simulink model "GunnerusDP_v1"  (R2017b)
settings: Solver=ode4  StartTime=0.0  StopTime=Tsim  FixedStep=ts  RelTol=1e-3  EnableMultiTasking=on
values from neighbouring files (symbols this model uses):
  ts = 0.01    [InitGunnerusDP.m]
undefined symbols (not defined in the file or in its folder): Control, Current, Hoerner, Par, Sim, TC_currentChange, vessel, vesselABC
libraries: marine_hydro x4, marine_gnc x3, simulink x3
(part 2 of 4)

== system GunnerusDP_v1/Environment and Vessel Dynamics/Wave definiton (from MCSim)/wave height and wave frequency/Hs and omega17 ==
  t : Inport
  Mux : Mux  Inputs=2
  hs : Subsystem  mask{v1=Par.Wave.hs(17), v2=Par.Wave.hs(18), t1=Par.Wave.time_change(33), t2=Par.Wave.time_change(34)}
      mask prompts: v1 "value1"; v2 "value2"; t1 "time1"; t2 "time2"
      mask Display:
      | plot([0 1 4 5], [0 0 4 4])
      | port_label('output', 1, 'y')
      | port_label('input', 1, 'time')
  omega_p : Subsystem  mask{v1=Par.Wave.omega_peak(17), v2=Par.Wave.omega_peak(18), t1=Par.Wave.time_change(33), t2=Par.Wave.time_change(34)}
      mask prompts: v1 "value1"; v2 "value2"; t1 "time1"; t2 "time2"
      mask Display:
      | plot([0 1 4 5], [0 0 4 4])
      | port_label('output', 1, 'y')
      | port_label('input', 1, 'time')
  Hs : Outport
  Hs n omega : Outport  Port=2
  wires:
  omega_p/1(omega_peak) -> Mux/2
  Mux/1 -> Hs n omega/1
  hs/1(omega_peak) -> Mux/1, Hs/1
  t/1 -> hs/1(time), omega_p/1(time)

== system GunnerusDP_v1/Environment and Vessel Dynamics/Wave definiton (from MCSim)/wave height and wave frequency/Hs and omega18 ==
  t : Inport
  Mux : Mux  Inputs=2
  hs : Subsystem  mask{v1=Par.Wave.hs(18), v2=Par.Wave.hs(19), t1=Par.Wave.time_change(35), t2=Par.Wave.time_change(36)}
      mask prompts: v1 "value1"; v2 "value2"; t1 "time1"; t2 "time2"
      mask Display:
      | plot([0 1 4 5], [0 0 4 4])
      | port_label('output', 1, 'y')
      | port_label('input', 1, 'time')
  omega_p : Subsystem  mask{v1=Par.Wave.omega_peak(18), v2=Par.Wave.omega_peak(19), t1=Par.Wave.time_change(35), t2=Par.Wave.time_change(36)}
      mask prompts: v1 "value1"; v2 "value2"; t1 "time1"; t2 "time2"
      mask Display:
      | plot([0 1 4 5], [0 0 4 4])
      | port_label('output', 1, 'y')
      | port_label('input', 1, 'time')
  Hs : Outport
  Hs n omega : Outport  Port=2
  wires:
  t/1 -> omega_p/1(time), hs/1(time)
  hs/1(omega_peak) -> Hs/1, Mux/1
  Mux/1 -> Hs n omega/1
  omega_p/1(omega_peak) -> Mux/2

== system GunnerusDP_v1/Environment and Vessel Dynamics/Wave definiton (from MCSim)/wave height and wave frequency/Hs and omega19 ==
  t : Inport
  Mux : Mux  Inputs=2
  hs : Subsystem  mask{v1=Par.Wave.hs(19), v2=Par.Wave.hs(20), t1=Par.Wave.time_change(37), t2=Par.Wave.time_change(38)}
      mask prompts: v1 "value1"; v2 "value2"; t1 "time1"; t2 "time2"
      mask Display:
      | plot([0 1 4 5], [0 0 4 4])
      | port_label('output', 1, 'y')
      | port_label('input', 1, 'time')
  omega_p : Subsystem  mask{v1=Par.Wave.omega_peak(19), v2=Par.Wave.omega_peak(20), t1=Par.Wave.time_change(37), t2=Par.Wave.time_change(38)}
      mask prompts: v1 "value1"; v2 "value2"; t1 "time1"; t2 "time2"
      mask Display:
      | plot([0 1 4 5], [0 0 4 4])
      | port_label('output', 1, 'y')
      | port_label('input', 1, 'time')
  Hs : Outport
  Hs n omega : Outport  Port=2
  wires:
  omega_p/1(omega_peak) -> Mux/2
  Mux/1 -> Hs n omega/1
  hs/1(omega_peak) -> Mux/1, Hs/1
  t/1 -> hs/1(time), omega_p/1(time)

== system GunnerusDP_v1/Environment and Vessel Dynamics/Wave definiton (from MCSim)/wave height and wave frequency/Hs and omega2 ==
  t : Inport
  Mux : Mux  Inputs=2
  hs : Subsystem  mask{v1=Par.Wave.hs(2), v2=Par.Wave.hs(3), t1=Par.Wave.time_change(3), t2=Par.Wave.time_change(4)}
      mask prompts: v1 "value1"; v2 "value2"; t1 "time1"; t2 "time2"
      mask Display:
      | plot([0 1 4 5], [0 0 4 4])
      | port_label('output', 1, 'y')
      | port_label('input', 1, 'time')
  omega_p : Subsystem  mask{v1=Par.Wave.omega_peak(2), v2=Par.Wave.omega_peak(3), t1=Par.Wave.time_change(3), t2=Par.Wave.time_change(4)}
      mask prompts: v1 "value1"; v2 "value2"; t1 "time1"; t2 "time2"
      mask Display:
      | plot([0 1 4 5], [0 0 4 4])
      | port_label('output', 1, 'y')
      | port_label('input', 1, 'time')
  Hs : Outport
  Hs n omega : Outport  Port=2
  wires:
  omega_p/1(omega_peak) -> Mux/2
  Mux/1 -> Hs n omega/1
  hs/1(omega_peak) -> Mux/1, Hs/1
  t/1 -> hs/1(time), omega_p/1(time)

== system GunnerusDP_v1/Environment and Vessel Dynamics/Wave definiton (from MCSim)/wave height and wave frequency/Hs and omega20 ==
  t : Inport
  Mux : Mux  Inputs=2
  hs : Subsystem  mask{v1=Par.Wave.hs(20), v2=Par.Wave.hs(21), t1=Par.Wave.time_change(39), t2=Par.Wave.time_change(40)}
      mask prompts: v1 "value1"; v2 "value2"; t1 "time1"; t2 "time2"
      mask Display:
      | plot([0 1 4 5], [0 0 4 4])
      | port_label('output', 1, 'y')
      | port_label('input', 1, 'time')
  omega_p : Subsystem  mask{v1=Par.Wave.omega_peak(20), v2=Par.Wave.omega_peak(21), t1=Par.Wave.time_change(39), t2=Par.Wave.time_change(40)}
      mask prompts: v1 "value1"; v2 "value2"; t1 "time1"; t2 "time2"
      mask Display:
      | plot([0 1 4 5], [0 0 4 4])
      | port_label('output', 1, 'y')
      | port_label('input', 1, 'time')
  Hs : Outport
  Hs n omega : Outport  Port=2
  wires:
  t/1 -> omega_p/1(time), hs/1(time)
  hs/1(omega_peak) -> Hs/1, Mux/1
  Mux/1 -> Hs n omega/1
  omega_p/1(omega_peak) -> Mux/2

== system GunnerusDP_v1/Environment and Vessel Dynamics/Wave definiton (from MCSim)/wave height and wave frequency/Hs and omega21 ==
  t : Inport
  Mux : Mux  Inputs=2
  hs : Subsystem  mask{v1=Par.Wave.hs(21), v2=Par.Wave.hs(22), t1=Par.Wave.time_change(41), t2=Par.Wave.time_change(42)}
      mask prompts: v1 "value1"; v2 "value2"; t1 "time1"; t2 "time2"
      mask Display:
      | plot([0 1 4 5], [0 0 4 4])
      | port_label('output', 1, 'y')
      | port_label('input', 1, 'time')
  omega_p : Subsystem  mask{v1=Par.Wave.omega_peak(21), v2=Par.Wave.omega_peak(22), t1=Par.Wave.time_change(41), t2=Par.Wave.time_change(42)}
      mask prompts: v1 "value1"; v2 "value2"; t1 "time1"; t2 "time2"
      mask Display:
      | plot([0 1 4 5], [0 0 4 4])
      | port_label('output', 1, 'y')
      | port_label('input', 1, 'time')
  Hs : Outport
  Hs n omega : Outport  Port=2
  wires:
  omega_p/1(omega_peak) -> Mux/2
  Mux/1 -> Hs n omega/1
  hs/1(omega_peak) -> Mux/1, Hs/1
  t/1 -> hs/1(time), omega_p/1(time)

== system GunnerusDP_v1/Environment and Vessel Dynamics/Wave definiton (from MCSim)/wave height and wave frequency/Hs and omega22 ==
  t : Inport
  Mux : Mux  Inputs=2
  hs : Subsystem  mask{v1=Par.Wave.hs(22), v2=Par.Wave.hs(23), t1=Par.Wave.time_change(43), t2=Par.Wave.time_change(44)}
      mask prompts: v1 "value1"; v2 "value2"; t1 "time1"; t2 "time2"
      mask Display:
      | plot([0 1 4 5], [0 0 4 4])
      | port_label('output', 1, 'y')
      | port_label('input', 1, 'time')
  omega_p : Subsystem  mask{v1=Par.Wave.omega_peak(22), v2=Par.Wave.omega_peak(23), t1=Par.Wave.time_change(43), t2=Par.Wave.time_change(44)}
      mask prompts: v1 "value1"; v2 "value2"; t1 "time1"; t2 "time2"
      mask Display:
      | plot([0 1 4 5], [0 0 4 4])
      | port_label('output', 1, 'y')
      | port_label('input', 1, 'time')
  Hs : Outport
  Hs n omega : Outport  Port=2
  wires:
  t/1 -> omega_p/1(time), hs/1(time)
  hs/1(omega_peak) -> Hs/1, Mux/1
  Mux/1 -> Hs n omega/1
  omega_p/1(omega_peak) -> Mux/2

== system GunnerusDP_v1/Environment and Vessel Dynamics/Wave definiton (from MCSim)/wave height and wave frequency/Hs and omega23 ==
  t : Inport
  Mux : Mux  Inputs=2
  hs : Subsystem  mask{v1=Par.Wave.hs(23), v2=Par.Wave.hs(24), t1=Par.Wave.time_change(45), t2=Par.Wave.time_change(46)}
      mask prompts: v1 "value1"; v2 "value2"; t1 "time1"; t2 "time2"
      mask Display:
      | plot([0 1 4 5], [0 0 4 4])
      | port_label('output', 1, 'y')
      | port_label('input', 1, 'time')
  omega_p : Subsystem  mask{v1=Par.Wave.omega_peak(23), v2=Par.Wave.omega_peak(24), t1=Par.Wave.time_change(45), t2=Par.Wave.time_change(46)}
      mask prompts: v1 "value1"; v2 "value2"; t1 "time1"; t2 "time2"
      mask Display:
      | plot([0 1 4 5], [0 0 4 4])
      | port_label('output', 1, 'y')
      | port_label('input', 1, 'time')
  Hs : Outport
  Hs n omega : Outport  Port=2
  wires:
  omega_p/1(omega_peak) -> Mux/2
  Mux/1 -> Hs n omega/1
  hs/1(omega_peak) -> Mux/1, Hs/1
  t/1 -> hs/1(time), omega_p/1(time)

== system GunnerusDP_v1/Environment and Vessel Dynamics/Wave definiton (from MCSim)/wave height and wave frequency/Hs and omega24 ==
  t : Inport
  Mux : Mux  Inputs=2
  hs : Subsystem  mask{v1=Par.Wave.hs(24), v2=Par.Wave.hs(25), t1=Par.Wave.time_change(47), t2=Par.Wave.time_change(48)}
      mask prompts: v1 "value1"; v2 "value2"; t1 "time1"; t2 "time2"
      mask Display:
      | plot([0 1 4 5], [0 0 4 4])
      | port_label('output', 1, 'y')
      | port_label('input', 1, 'time')
  omega_p : Subsystem  mask{v1=Par.Wave.omega_peak(24), v2=Par.Wave.omega_peak(25), t1=Par.Wave.time_change(47), t2=Par.Wave.time_change(48)}
      mask prompts: v1 "value1"; v2 "value2"; t1 "time1"; t2 "time2"
      mask Display:
      | plot([0 1 4 5], [0 0 4 4])
      | port_label('output', 1, 'y')
      | port_label('input', 1, 'time')
  Hs : Outport
  Hs n omega : Outport  Port=2
  wires:
  t/1 -> omega_p/1(time), hs/1(time)
  hs/1(omega_peak) -> Hs/1, Mux/1
  Mux/1 -> Hs n omega/1
  omega_p/1(omega_peak) -> Mux/2

== system GunnerusDP_v1/Environment and Vessel Dynamics/Wave definiton (from MCSim)/wave height and wave frequency/Hs and omega3 ==
  t : Inport
  Mux : Mux  Inputs=2
  hs : Subsystem  mask{v1=Par.Wave.hs(3), v2=Par.Wave.hs(4), t1=Par.Wave.time_change(5), t2=Par.Wave.time_change(6)}
      mask prompts: v1 "value1"; v2 "value2"; t1 "time1"; t2 "time2"
      mask Display:
      | plot([0 1 4 5], [0 0 4 4])
      | port_label('output', 1, 'y')
      | port_label('input', 1, 'time')
  omega_p : Subsystem  mask{v1=Par.Wave.omega_peak(3), v2=Par.Wave.omega_peak(4), t1=Par.Wave.time_change(5), t2=Par.Wave.time_change(6)}
      mask prompts: v1 "value1"; v2 "value2"; t1 "time1"; t2 "time2"
      mask Display:
      | plot([0 1 4 5], [0 0 4 4])
      | port_label('output', 1, 'y')
      | port_label('input', 1, 'time')
  Hs : Outport
  Hs n omega : Outport  Port=2
  wires:
  t/1 -> omega_p/1(time), hs/1(time)
  hs/1(omega_peak) -> Hs/1, Mux/1
  Mux/1 -> Hs n omega/1
  omega_p/1(omega_peak) -> Mux/2

== system GunnerusDP_v1/Environment and Vessel Dynamics/Wave definiton (from MCSim)/wave height and wave frequency/Hs and omega4 ==
  t : Inport
  Mux : Mux  Inputs=2
  hs : Subsystem  mask{v1=Par.Wave.hs(4), v2=Par.Wave.hs(5), t1=Par.Wave.time_change(7), t2=Par.Wave.time_change(8)}
      mask prompts: v1 "value1"; v2 "value2"; t1 "time1"; t2 "time2"
      mask Display:
      | plot([0 1 4 5], [0 0 4 4])
      | port_label('output', 1, 'y')
      | port_label('input', 1, 'time')
  omega_p : Subsystem  mask{v1=Par.Wave.omega_peak(4), v2=Par.Wave.omega_peak(5), t1=Par.Wave.time_change(7), t2=Par.Wave.time_change(8)}
      mask prompts: v1 "value1"; v2 "value2"; t1 "time1"; t2 "time2"
      mask Display:
      | plot([0 1 4 5], [0 0 4 4])
      | port_label('output', 1, 'y')
      | port_label('input', 1, 'time')
  Hs : Outport
  Hs n omega : Outport  Port=2
  wires:
  omega_p/1(omega_peak) -> Mux/2
  Mux/1 -> Hs n omega/1
  hs/1(omega_peak) -> Mux/1, Hs/1
  t/1 -> hs/1(time), omega_p/1(time)

== system GunnerusDP_v1/Environment and Vessel Dynamics/Wave definiton (from MCSim)/wave height and wave frequency/Hs and omega5 ==
  t : Inport
  Mux : Mux  Inputs=2
  hs : Subsystem  mask{v1=Par.Wave.hs(5), v2=Par.Wave.hs(6), t1=Par.Wave.time_change(9), t2=Par.Wave.time_change(10)}
      mask prompts: v1 "value1"; v2 "value2"; t1 "time1"; t2 "time2"
      mask Display:
      | plot([0 1 4 5], [0 0 4 4])
      | port_label('output', 1, 'y')
      | port_label('input', 1, 'time')
  omega_p : Subsystem  mask{v1=Par.Wave.omega_peak(5), v2=Par.Wave.omega_peak(6), t1=Par.Wave.time_change(9), t2=Par.Wave.time_change(10)}
      mask prompts: v1 "value1"; v2 "value2"; t1 "time1"; t2 "time2"
      mask Display:
      | plot([0 1 4 5], [0 0 4 4])
      | port_label('output', 1, 'y')
      | port_label('input', 1, 'time')
  Hs : Outport
  Hs n omega : Outport  Port=2
  wires:
  t/1 -> omega_p/1(time), hs/1(time)
  hs/1(omega_peak) -> Hs/1, Mux/1
  Mux/1 -> Hs n omega/1
  omega_p/1(omega_peak) -> Mux/2

== system GunnerusDP_v1/Environment and Vessel Dynamics/Wave definiton (from MCSim)/wave height and wave frequency/Hs and omega6 ==
  t : Inport
  Mux : Mux  Inputs=2
  hs : Subsystem  mask{v1=Par.Wave.hs(6), v2=Par.Wave.hs(7), t1=Par.Wave.time_change(11), t2=Par.Wave.time_change(12)}
      mask prompts: v1 "value1"; v2 "value2"; t1 "time1"; t2 "time2"
      mask Display:
      | plot([0 1 4 5], [0 0 4 4])
      | port_label('output', 1, 'y')
      | port_label('input', 1, 'time')
  omega_p : Subsystem  mask{v1=Par.Wave.omega_peak(6), v2=Par.Wave.omega_peak(7), t1=Par.Wave.time_change(11), t2=Par.Wave.time_change(12)}
      mask prompts: v1 "value1"; v2 "value2"; t1 "time1"; t2 "time2"
      mask Display:
      | plot([0 1 4 5], [0 0 4 4])
      | port_label('output', 1, 'y')
      | port_label('input', 1, 'time')
  Hs : Outport
  Hs n omega : Outport  Port=2
  wires:
  omega_p/1(omega_peak) -> Mux/2
  Mux/1 -> Hs n omega/1
  hs/1(omega_peak) -> Mux/1, Hs/1
  t/1 -> hs/1(time), omega_p/1(time)

== system GunnerusDP_v1/Environment and Vessel Dynamics/Wave definiton (from MCSim)/wave height and wave frequency/Hs and omega7 ==
  t : Inport
  Mux : Mux  Inputs=2
  hs : Subsystem  mask{v1=Par.Wave.hs(7), v2=Par.Wave.hs(8), t1=Par.Wave.time_change(13), t2=Par.Wave.time_change(14)}
      mask prompts: v1 "value1"; v2 "value2"; t1 "time1"; t2 "time2"
      mask Display:
      | plot([0 1 4 5], [0 0 4 4])
      | port_label('output', 1, 'y')
      | port_label('input', 1, 'time')
  omega_p : Subsystem  mask{v1=Par.Wave.omega_peak(7), v2=Par.Wave.omega_peak(8), t1=Par.Wave.time_change(13), t2=Par.Wave.time_change(14)}
      mask prompts: v1 "value1"; v2 "value2"; t1 "time1"; t2 "time2"
      mask Display:
      | plot([0 1 4 5], [0 0 4 4])
      | port_label('output', 1, 'y')
      | port_label('input', 1, 'time')
  Hs : Outport
  Hs n omega : Outport  Port=2
  wires:
  t/1 -> omega_p/1(time), hs/1(time)
  hs/1(omega_peak) -> Hs/1, Mux/1
  Mux/1 -> Hs n omega/1
  omega_p/1(omega_peak) -> Mux/2

== system GunnerusDP_v1/Environment and Vessel Dynamics/Wave definiton (from MCSim)/wave height and wave frequency/Hs and omega8 ==
  t : Inport
  Mux : Mux  Inputs=2
  hs : Subsystem  mask{v1=Par.Wave.hs(8), v2=Par.Wave.hs(9), t1=Par.Wave.time_change(15), t2=Par.Wave.time_change(16)}
      mask prompts: v1 "value1"; v2 "value2"; t1 "time1"; t2 "time2"
      mask Display:
      | plot([0 1 4 5], [0 0 4 4])
      | port_label('output', 1, 'y')
      | port_label('input', 1, 'time')
  omega_p : Subsystem  mask{v1=Par.Wave.omega_peak(8), v2=Par.Wave.omega_peak(9), t1=Par.Wave.time_change(15), t2=Par.Wave.time_change(16)}
      mask prompts: v1 "value1"; v2 "value2"; t1 "time1"; t2 "time2"
      mask Display:
      | plot([0 1 4 5], [0 0 4 4])
      | port_label('output', 1, 'y')
      | port_label('input', 1, 'time')
  Hs : Outport
  Hs n omega : Outport  Port=2
  wires:
  omega_p/1(omega_peak) -> Mux/2
  Mux/1 -> Hs n omega/1
  hs/1(omega_peak) -> Mux/1, Hs/1
  t/1 -> hs/1(time), omega_p/1(time)

== system GunnerusDP_v1/Environment and Vessel Dynamics/Wave definiton (from MCSim)/wave height and wave frequency/Hs and omega9 ==
  t : Inport
  Mux : Mux  Inputs=2
  hs : Subsystem  mask{v1=Par.Wave.hs(9), v2=Par.Wave.hs(10), t1=Par.Wave.time_change(17), t2=Par.Wave.time_change(18)}
      mask prompts: v1 "value1"; v2 "value2"; t1 "time1"; t2 "time2"
      mask Display:
      | plot([0 1 4 5], [0 0 4 4])
      | port_label('output', 1, 'y')
      | port_label('input', 1, 'time')
  omega_p : Subsystem  mask{v1=Par.Wave.omega_peak(9), v2=Par.Wave.omega_peak(10), t1=Par.Wave.time_change(17), t2=Par.Wave.time_change(18)}
      mask prompts: v1 "value1"; v2 "value2"; t1 "time1"; t2 "time2"
      mask Display:
      | plot([0 1 4 5], [0 0 4 4])
      | port_label('output', 1, 'y')
      | port_label('input', 1, 'time')
  Hs : Outport
  Hs n omega : Outport  Port=2
  wires:
  t/1 -> omega_p/1(time), hs/1(time)
  hs/1(omega_peak) -> Hs/1, Mux/1
  Mux/1 -> Hs n omega/1
  omega_p/1(omega_peak) -> Mux/2

== system GunnerusDP_v1/Environment and Vessel Dynamics/Wave definiton (from MCSim)/wave height and wave frequency/Count/switch1 ==
  hs : Inport
  Constant : Constant  Value=a
  Gain : Gain  Gain=1/(b-a)  SaturateOnIntegerOverflow=on  OutDataTypeStr=Inherit: Same as input  ParamDataTypeStr=Inherit: Same as input
  Sum : Sum  Inputs=-+  SaturateOnIntegerOverflow=on
  switch : Outport
  wires:
  Constant/1 -> Sum/1
  Sum/1 -> Gain/1
  Gain/1 -> switch/1
  hs/1 -> Sum/2

== system GunnerusDP_v1/Environment and Vessel Dynamics/Wave definiton (from MCSim)/wave height and wave frequency/Count/switch10 ==
  hs : Inport
  Constant : Constant  Value=a
  Gain : Gain  Gain=1/(b-a)  SaturateOnIntegerOverflow=on  OutDataTypeStr=Inherit: Same as input  ParamDataTypeStr=Inherit: Same as input
  Sum : Sum  Inputs=-+  SaturateOnIntegerOverflow=on
  switch : Outport
  wires:
  hs/1 -> Sum/2
  Gain/1 -> switch/1
  Sum/1 -> Gain/1
  Constant/1 -> Sum/1

== system GunnerusDP_v1/Environment and Vessel Dynamics/Wave definiton (from MCSim)/wave height and wave frequency/Count/switch11 ==
  hs : Inport
  Constant : Constant  Value=a
  Gain : Gain  Gain=1/(b-a)  SaturateOnIntegerOverflow=on  OutDataTypeStr=Inherit: Same as input  ParamDataTypeStr=Inherit: Same as input
  Sum : Sum  Inputs=-+  SaturateOnIntegerOverflow=on
  switch : Outport
  wires:
  hs/1 -> Sum/2
  Gain/1 -> switch/1
  Sum/1 -> Gain/1
  Constant/1 -> Sum/1

== system GunnerusDP_v1/Environment and Vessel Dynamics/Wave definiton (from MCSim)/wave height and wave frequency/Count/switch12 ==
  hs : Inport
  Constant : Constant  Value=a
  Gain : Gain  Gain=1/(b-a)  SaturateOnIntegerOverflow=on  OutDataTypeStr=Inherit: Same as input  ParamDataTypeStr=Inherit: Same as input
  Sum : Sum  Inputs=-+  SaturateOnIntegerOverflow=on
  switch : Outport
  wires:
  hs/1 -> Sum/2
  Gain/1 -> switch/1
  Sum/1 -> Gain/1
  Constant/1 -> Sum/1

== system GunnerusDP_v1/Environment and Vessel Dynamics/Wave definiton (from MCSim)/wave height and wave frequency/Count/switch13 ==
  hs : Inport
  Constant : Constant  Value=a
  Gain : Gain  Gain=1/(b-a)  SaturateOnIntegerOverflow=on  OutDataTypeStr=Inherit: Same as input  ParamDataTypeStr=Inherit: Same as input
  Sum : Sum  Inputs=-+  SaturateOnIntegerOverflow=on
  switch : Outport
  wires:
  hs/1 -> Sum/2
  Gain/1 -> switch/1
  Sum/1 -> Gain/1
  Constant/1 -> Sum/1

== system GunnerusDP_v1/Environment and Vessel Dynamics/Wave definiton (from MCSim)/wave height and wave frequency/Count/switch14 ==
  hs : Inport
  Constant : Constant  Value=a
  Gain : Gain  Gain=1/(b-a)  SaturateOnIntegerOverflow=on  OutDataTypeStr=Inherit: Same as input  ParamDataTypeStr=Inherit: Same as input
  Sum : Sum  Inputs=-+  SaturateOnIntegerOverflow=on
  switch : Outport
  wires:
  hs/1 -> Sum/2
  Gain/1 -> switch/1
  Sum/1 -> Gain/1
  Constant/1 -> Sum/1

== system GunnerusDP_v1/Environment and Vessel Dynamics/Wave definiton (from MCSim)/wave height and wave frequency/Count/switch15 ==
  hs : Inport
  Constant : Constant  Value=a
  Gain : Gain  Gain=1/(b-a)  SaturateOnIntegerOverflow=on  OutDataTypeStr=Inherit: Same as input  ParamDataTypeStr=Inherit: Same as input
  Sum : Sum  Inputs=-+  SaturateOnIntegerOverflow=on
  switch : Outport
  wires:
  hs/1 -> Sum/2
  Gain/1 -> switch/1
  Sum/1 -> Gain/1
  Constant/1 -> Sum/1

== system GunnerusDP_v1/Environment and Vessel Dynamics/Wave definiton (from MCSim)/wave height and wave frequency/Count/switch16 ==
  hs : Inport
  Constant : Constant  Value=a
  Gain : Gain  Gain=1/(b-a)  SaturateOnIntegerOverflow=on  OutDataTypeStr=Inherit: Same as input  ParamDataTypeStr=Inherit: Same as input
  Sum : Sum  Inputs=-+  SaturateOnIntegerOverflow=on
  switch : Outport
  wires:
  hs/1 -> Sum/2
  Gain/1 -> switch/1
  Sum/1 -> Gain/1
  Constant/1 -> Sum/1

== system GunnerusDP_v1/Environment and Vessel Dynamics/Wave definiton (from MCSim)/wave height and wave frequency/Count/switch17 ==
  hs : Inport
  Constant : Constant  Value=a
  Gain : Gain  Gain=1/(b-a)  SaturateOnIntegerOverflow=on  OutDataTypeStr=Inherit: Same as input  ParamDataTypeStr=Inherit: Same as input
  Sum : Sum  Inputs=-+  SaturateOnIntegerOverflow=on
  switch : Outport
  wires:
  Constant/1 -> Sum/1
  Sum/1 -> Gain/1
  Gain/1 -> switch/1
  hs/1 -> Sum/2

== system GunnerusDP_v1/Environment and Vessel Dynamics/Wave definiton (from MCSim)/wave height and wave frequency/Count/switch18 ==
  hs : Inport
  Constant : Constant  Value=a
  Gain : Gain  Gain=1/(b-a)  SaturateOnIntegerOverflow=on  OutDataTypeStr=Inherit: Same as input  ParamDataTypeStr=Inherit: Same as input
  Sum : Sum  Inputs=-+  SaturateOnIntegerOverflow=on
  switch : Outport
  wires:
  hs/1 -> Sum/2
  Gain/1 -> switch/1
  Sum/1 -> Gain/1
  Constant/1 -> Sum/1

== system GunnerusDP_v1/Environment and Vessel Dynamics/Wave definiton (from MCSim)/wave height and wave frequency/Count/switch19 ==
  hs : Inport
  Constant : Constant  Value=a
  Gain : Gain  Gain=1/(b-a)  SaturateOnIntegerOverflow=on  OutDataTypeStr=Inherit: Same as input  ParamDataTypeStr=Inherit: Same as input
  Sum : Sum  Inputs=-+  SaturateOnIntegerOverflow=on
  switch : Outport
  wires:
  hs/1 -> Sum/2
  Gain/1 -> switch/1
  Sum/1 -> Gain/1
  Constant/1 -> Sum/1

== system GunnerusDP_v1/Environment and Vessel Dynamics/Wave definiton (from MCSim)/wave height and wave frequency/Count/switch2 ==
  hs : Inport
  Constant : Constant  Value=a
  Gain : Gain  Gain=1/(b-a)  SaturateOnIntegerOverflow=on  OutDataTypeStr=Inherit: Same as input  ParamDataTypeStr=Inherit: Same as input
  Sum : Sum  Inputs=-+  SaturateOnIntegerOverflow=on
  switch : Outport
  wires:
  hs/1 -> Sum/2
  Gain/1 -> switch/1
  Sum/1 -> Gain/1
  Constant/1 -> Sum/1

== system GunnerusDP_v1/Environment and Vessel Dynamics/Wave definiton (from MCSim)/wave height and wave frequency/Count/switch20 ==
  hs : Inport
  Constant : Constant  Value=a
  Gain : Gain  Gain=1/(b-a)  SaturateOnIntegerOverflow=on  OutDataTypeStr=Inherit: Same as input  ParamDataTypeStr=Inherit: Same as input
  Sum : Sum  Inputs=-+  SaturateOnIntegerOverflow=on
  switch : Outport
  wires:
  hs/1 -> Sum/2
  Gain/1 -> switch/1
  Sum/1 -> Gain/1
  Constant/1 -> Sum/1

== system GunnerusDP_v1/Environment and Vessel Dynamics/Wave definiton (from MCSim)/wave height and wave frequency/Count/switch21 ==
  hs : Inport
  Constant : Constant  Value=a
  Gain : Gain  Gain=1/(b-a)  SaturateOnIntegerOverflow=on  OutDataTypeStr=Inherit: Same as input  ParamDataTypeStr=Inherit: Same as input
  Sum : Sum  Inputs=-+  SaturateOnIntegerOverflow=on
  switch : Outport
  wires:
  hs/1 -> Sum/2
  Gain/1 -> switch/1
  Sum/1 -> Gain/1
  Constant/1 -> Sum/1

== system GunnerusDP_v1/Environment and Vessel Dynamics/Wave definiton (from MCSim)/wave height and wave frequency/Count/switch22 ==
  hs : Inport
  Constant : Constant  Value=a
  Gain : Gain  Gain=1/(b-a)  SaturateOnIntegerOverflow=on  OutDataTypeStr=Inherit: Same as input  ParamDataTypeStr=Inherit: Same as input
  Sum : Sum  Inputs=-+  SaturateOnIntegerOverflow=on
  switch : Outport
  wires:
  hs/1 -> Sum/2
  Gain/1 -> switch/1
  Sum/1 -> Gain/1
  Constant/1 -> Sum/1

== system GunnerusDP_v1/Environment and Vessel Dynamics/Wave definiton (from MCSim)/wave height and wave frequency/Count/switch23 ==
  hs : Inport
  Constant : Constant  Value=a
  Gain : Gain  Gain=1/(b-a)  SaturateOnIntegerOverflow=on  OutDataTypeStr=Inherit: Same as input  ParamDataTypeStr=Inherit: Same as input
  Sum : Sum  Inputs=-+  SaturateOnIntegerOverflow=on
  switch : Outport
  wires:
  hs/1 -> Sum/2
  Gain/1 -> switch/1
  Sum/1 -> Gain/1
  Constant/1 -> Sum/1

== system GunnerusDP_v1/Environment and Vessel Dynamics/Wave definiton (from MCSim)/wave height and wave frequency/Count/switch3 ==
  hs : Inport
  Constant : Constant  Value=a
  Gain : Gain  Gain=1/(b-a)  SaturateOnIntegerOverflow=on  OutDataTypeStr=Inherit: Same as input  ParamDataTypeStr=Inherit: Same as input
  Sum : Sum  Inputs=-+  SaturateOnIntegerOverflow=on
  switch : Outport
  wires:
  hs/1 -> Sum/2
  Gain/1 -> switch/1
  Sum/1 -> Gain/1
  Constant/1 -> Sum/1

== system GunnerusDP_v1/Environment and Vessel Dynamics/Wave definiton (from MCSim)/wave height and wave frequency/Count/switch4 ==
  hs : Inport
  Constant : Constant  Value=a
  Gain : Gain  Gain=1/(b-a)  SaturateOnIntegerOverflow=on  OutDataTypeStr=Inherit: Same as input  ParamDataTypeStr=Inherit: Same as input
  Sum : Sum  Inputs=-+  SaturateOnIntegerOverflow=on
  switch : Outport
  wires:
  hs/1 -> Sum/2
  Gain/1 -> switch/1
  Sum/1 -> Gain/1
  Constant/1 -> Sum/1

== system GunnerusDP_v1/Environment and Vessel Dynamics/Wave definiton (from MCSim)/wave height and wave frequency/Count/switch5 ==
  hs : Inport
  Constant : Constant  Value=a
  Gain : Gain  Gain=1/(b-a)  SaturateOnIntegerOverflow=on  OutDataTypeStr=Inherit: Same as input  ParamDataTypeStr=Inherit: Same as input
  Sum : Sum  Inputs=-+  SaturateOnIntegerOverflow=on
  switch : Outport
  wires:
  hs/1 -> Sum/2
  Gain/1 -> switch/1
  Sum/1 -> Gain/1
  Constant/1 -> Sum/1

== system GunnerusDP_v1/Environment and Vessel Dynamics/Wave definiton (from MCSim)/wave height and wave frequency/Count/switch6 ==
  hs : Inport
  Constant : Constant  Value=a
  Gain : Gain  Gain=1/(b-a)  SaturateOnIntegerOverflow=on  OutDataTypeStr=Inherit: Same as input  ParamDataTypeStr=Inherit: Same as input
  Sum : Sum  Inputs=-+  SaturateOnIntegerOverflow=on
  switch : Outport
  wires:
  hs/1 -> Sum/2
  Gain/1 -> switch/1
  Sum/1 -> Gain/1
  Constant/1 -> Sum/1

== system GunnerusDP_v1/Environment and Vessel Dynamics/Wave definiton (from MCSim)/wave height and wave frequency/Count/switch7 ==
  hs : Inport
  Constant : Constant  Value=a
  Gain : Gain  Gain=1/(b-a)  SaturateOnIntegerOverflow=on  OutDataTypeStr=Inherit: Same as input  ParamDataTypeStr=Inherit: Same as input
  Sum : Sum  Inputs=-+  SaturateOnIntegerOverflow=on
  switch : Outport
  wires:
  hs/1 -> Sum/2
  Gain/1 -> switch/1
  Sum/1 -> Gain/1
  Constant/1 -> Sum/1

== system GunnerusDP_v1/Environment and Vessel Dynamics/Wave definiton (from MCSim)/wave height and wave frequency/Count/switch8 ==
  hs : Inport
  Constant : Constant  Value=a
  Gain : Gain  Gain=1/(b-a)  SaturateOnIntegerOverflow=on  OutDataTypeStr=Inherit: Same as input  ParamDataTypeStr=Inherit: Same as input
  Sum : Sum  Inputs=-+  SaturateOnIntegerOverflow=on
  switch : Outport
  wires:
  hs/1 -> Sum/2
  Gain/1 -> switch/1
  Sum/1 -> Gain/1
  Constant/1 -> Sum/1

== system GunnerusDP_v1/Environment and Vessel Dynamics/Wave definiton (from MCSim)/wave height and wave frequency/Count/switch9 ==
  hs : Inport
  Constant : Constant  Value=a
  Gain : Gain  Gain=1/(b-a)  SaturateOnIntegerOverflow=on  OutDataTypeStr=Inherit: Same as input  ParamDataTypeStr=Inherit: Same as input
  Sum : Sum  Inputs=-+  SaturateOnIntegerOverflow=on
  switch : Outport
  wires:
  Constant/1 -> Sum/1
  Sum/1 -> Gain/1
  Gain/1 -> switch/1
  hs/1 -> Sum/2

== system GunnerusDP_v1/Environment and Vessel Dynamics/Wave definiton (from MCSim)/wave height and wave frequency/Hs and omega1/hs ==
  time : Inport
  Constant : Constant  Value=v1
  Constant2 : Constant  Value=v2
  If : If  IfExpression=u1 < t1  ElseIfExpressions=u1>=t1 & u1<t2
  If Action Subsystem1 : Subsystem  TreatAsAtomicUnit=on
  If Action Subsystem2 : Subsystem  TreatAsAtomicUnit=on
  If Action Subsystem3 : Subsystem  TreatAsAtomicUnit=on
  Merge : Merge  Inputs=3
  omega_peak : Outport
  wires:
  time/1 -> If Action Subsystem2/1(In1), If/1
  If/3 -> If Action Subsystem3/Action
  If/1 -> If Action Subsystem1/Action
  Constant/1 -> If Action Subsystem1/1(In1)
  Constant2/1 -> If Action Subsystem3/1(In1)
  If Action Subsystem3/1(Out1) -> Merge/3
  If Action Subsystem2/1(Out1) -> Merge/2
  If/2 -> If Action Subsystem2/Action
  If Action Subsystem1/1(Out1) -> Merge/1
  Merge/1 -> omega_peak/1

== system GunnerusDP_v1/Environment and Vessel Dynamics/Wave definiton (from MCSim)/wave height and wave frequency/Hs and omega1/omega_p ==
  time : Inport
  Constant : Constant  Value=v1
  Constant2 : Constant  Value=v2
  If : If  IfExpression=u1 < t1  ElseIfExpressions=u1>=t1 & u1<t2
  If Action Subsystem1 : Subsystem  TreatAsAtomicUnit=on
  If Action Subsystem2 : Subsystem  TreatAsAtomicUnit=on
  If Action Subsystem3 : Subsystem  TreatAsAtomicUnit=on
  Merge : Merge  Inputs=3
  omega_peak : Outport
  wires:
  Merge/1 -> omega_peak/1
  If Action Subsystem1/1(Out1) -> Merge/1
  If/2 -> If Action Subsystem2/Action
  If Action Subsystem2/1(Out1) -> Merge/2
  If Action Subsystem3/1(Out1) -> Merge/3
  Constant2/1 -> If Action Subsystem3/1(In1)
  Constant/1 -> If Action Subsystem1/1(In1)
  If/1 -> If Action Subsystem1/Action
  If/3 -> If Action Subsystem3/Action
  time/1 -> If/1, If Action Subsystem2/1(In1)

== system GunnerusDP_v1/Environment and Vessel Dynamics/Wave definiton (from MCSim)/wave height and wave frequency/Hs and omega10/hs ==
  time : Inport
  Constant : Constant  Value=v1
  Constant2 : Constant  Value=v2
  If : If  IfExpression=u1 < t1  ElseIfExpressions=u1>=t1 & u1<t2
  If Action Subsystem1 : Subsystem  TreatAsAtomicUnit=on
  If Action Subsystem2 : Subsystem  TreatAsAtomicUnit=on
  If Action Subsystem3 : Subsystem  TreatAsAtomicUnit=on
  Merge : Merge  Inputs=3
  omega_peak : Outport
  wires:
  Merge/1 -> omega_peak/1
  If Action Subsystem1/1(Out1) -> Merge/1
  If/2 -> If Action Subsystem2/Action
  If Action Subsystem2/1(Out1) -> Merge/2
  If Action Subsystem3/1(Out1) -> Merge/3
  Constant2/1 -> If Action Subsystem3/1(In1)
  Constant/1 -> If Action Subsystem1/1(In1)
  If/1 -> If Action Subsystem1/Action
  If/3 -> If Action Subsystem3/Action
  time/1 -> If/1, If Action Subsystem2/1(In1)

== system GunnerusDP_v1/Environment and Vessel Dynamics/Wave definiton (from MCSim)/wave height and wave frequency/Hs and omega10/omega_p ==
  time : Inport
  Constant : Constant  Value=v1
  Constant2 : Constant  Value=v2
  If : If  IfExpression=u1 < t1  ElseIfExpressions=u1>=t1 & u1<t2
  If Action Subsystem1 : Subsystem  TreatAsAtomicUnit=on
  If Action Subsystem2 : Subsystem  TreatAsAtomicUnit=on
  If Action Subsystem3 : Subsystem  TreatAsAtomicUnit=on
  Merge : Merge  Inputs=3
  omega_peak : Outport
  wires:
  time/1 -> If Action Subsystem2/1(In1), If/1
  If/3 -> If Action Subsystem3/Action
  If/1 -> If Action Subsystem1/Action
  Constant/1 -> If Action Subsystem1/1(In1)
  Constant2/1 -> If Action Subsystem3/1(In1)
  If Action Subsystem3/1(Out1) -> Merge/3
  If Action Subsystem2/1(Out1) -> Merge/2
  If/2 -> If Action Subsystem2/Action
  If Action Subsystem1/1(Out1) -> Merge/1
  Merge/1 -> omega_peak/1

== system GunnerusDP_v1/Environment and Vessel Dynamics/Wave definiton (from MCSim)/wave height and wave frequency/Hs and omega11/hs ==
  time : Inport
  Constant : Constant  Value=v1
  Constant2 : Constant  Value=v2
  If : If  IfExpression=u1 < t1  ElseIfExpressions=u1>=t1 & u1<t2
  If Action Subsystem1 : Subsystem  TreatAsAtomicUnit=on
  If Action Subsystem2 : Subsystem  TreatAsAtomicUnit=on
  If Action Subsystem3 : Subsystem  TreatAsAtomicUnit=on
  Merge : Merge  Inputs=3
  omega_peak : Outport
  wires:
  time/1 -> If Action Subsystem2/1(In1), If/1
  If/3 -> If Action Subsystem3/Action
  If/1 -> If Action Subsystem1/Action
  Constant/1 -> If Action Subsystem1/1(In1)
  Constant2/1 -> If Action Subsystem3/1(In1)
  If Action Subsystem3/1(Out1) -> Merge/3
  If Action Subsystem2/1(Out1) -> Merge/2
  If/2 -> If Action Subsystem2/Action
  If Action Subsystem1/1(Out1) -> Merge/1
  Merge/1 -> omega_peak/1

== system GunnerusDP_v1/Environment and Vessel Dynamics/Wave definiton (from MCSim)/wave height and wave frequency/Hs and omega11/omega_p ==
  time : Inport
  Constant : Constant  Value=v1
  Constant2 : Constant  Value=v2
  If : If  IfExpression=u1 < t1  ElseIfExpressions=u1>=t1 & u1<t2
  If Action Subsystem1 : Subsystem  TreatAsAtomicUnit=on
  If Action Subsystem2 : Subsystem  TreatAsAtomicUnit=on
  If Action Subsystem3 : Subsystem  TreatAsAtomicUnit=on
  Merge : Merge  Inputs=3
  omega_peak : Outport
  wires:
  Merge/1 -> omega_peak/1
  If Action Subsystem1/1(Out1) -> Merge/1
  If/2 -> If Action Subsystem2/Action
  If Action Subsystem2/1(Out1) -> Merge/2
  If Action Subsystem3/1(Out1) -> Merge/3
  Constant2/1 -> If Action Subsystem3/1(In1)
  Constant/1 -> If Action Subsystem1/1(In1)
  If/1 -> If Action Subsystem1/Action
  If/3 -> If Action Subsystem3/Action
  time/1 -> If/1, If Action Subsystem2/1(In1)

== system GunnerusDP_v1/Environment and Vessel Dynamics/Wave definiton (from MCSim)/wave height and wave frequency/Hs and omega12/hs ==
  time : Inport
  Constant : Constant  Value=v1
  Constant2 : Constant  Value=v2
  If : If  IfExpression=u1 < t1  ElseIfExpressions=u1>=t1 & u1<t2
  If Action Subsystem1 : Subsystem  TreatAsAtomicUnit=on
  If Action Subsystem2 : Subsystem  TreatAsAtomicUnit=on
  If Action Subsystem3 : Subsystem  TreatAsAtomicUnit=on
  Merge : Merge  Inputs=3
  omega_peak : Outport
  wires:
  Merge/1 -> omega_peak/1
  If Action Subsystem1/1(Out1) -> Merge/1
  If/2 -> If Action Subsystem2/Action
  If Action Subsystem2/1(Out1) -> Merge/2
  If Action Subsystem3/1(Out1) -> Merge/3
  Constant2/1 -> If Action Subsystem3/1(In1)
  Constant/1 -> If Action Subsystem1/1(In1)
  If/1 -> If Action Subsystem1/Action
  If/3 -> If Action Subsystem3/Action
  time/1 -> If/1, If Action Subsystem2/1(In1)

== system GunnerusDP_v1/Environment and Vessel Dynamics/Wave definiton (from MCSim)/wave height and wave frequency/Hs and omega12/omega_p ==
  time : Inport
  Constant : Constant  Value=v1
  Constant2 : Constant  Value=v2
  If : If  IfExpression=u1 < t1  ElseIfExpressions=u1>=t1 & u1<t2
  If Action Subsystem1 : Subsystem  TreatAsAtomicUnit=on
  If Action Subsystem2 : Subsystem  TreatAsAtomicUnit=on
  If Action Subsystem3 : Subsystem  TreatAsAtomicUnit=on
  Merge : Merge  Inputs=3
  omega_peak : Outport
  wires:
  time/1 -> If Action Subsystem2/1(In1), If/1
  If/3 -> If Action Subsystem3/Action
  If/1 -> If Action Subsystem1/Action
  Constant/1 -> If Action Subsystem1/1(In1)
  Constant2/1 -> If Action Subsystem3/1(In1)
  If Action Subsystem3/1(Out1) -> Merge/3
  If Action Subsystem2/1(Out1) -> Merge/2
  If/2 -> If Action Subsystem2/Action
  If Action Subsystem1/1(Out1) -> Merge/1
  Merge/1 -> omega_peak/1

== system GunnerusDP_v1/Environment and Vessel Dynamics/Wave definiton (from MCSim)/wave height and wave frequency/Hs and omega13/hs ==
  time : Inport
  Constant : Constant  Value=v1
  Constant2 : Constant  Value=v2
  If : If  IfExpression=u1 < t1  ElseIfExpressions=u1>=t1 & u1<t2
  If Action Subsystem1 : Subsystem  TreatAsAtomicUnit=on
  If Action Subsystem2 : Subsystem  TreatAsAtomicUnit=on
  If Action Subsystem3 : Subsystem  TreatAsAtomicUnit=on
  Merge : Merge  Inputs=3
  omega_peak : Outport
  wires:
  time/1 -> If Action Subsystem2/1(In1), If/1
  If/3 -> If Action Subsystem3/Action
  If/1 -> If Action Subsystem1/Action
  Constant/1 -> If Action Subsystem1/1(In1)
  Constant2/1 -> If Action Subsystem3/1(In1)
  If Action Subsystem3/1(Out1) -> Merge/3
  If Action Subsystem2/1(Out1) -> Merge/2
  If/2 -> If Action Subsystem2/Action
  If Action Subsystem1/1(Out1) -> Merge/1
  Merge/1 -> omega_peak/1

== system GunnerusDP_v1/Environment and Vessel Dynamics/Wave definiton (from MCSim)/wave height and wave frequency/Hs and omega13/omega_p ==
  time : Inport
  Constant : Constant  Value=v1
  Constant2 : Constant  Value=v2
  If : If  IfExpression=u1 < t1  ElseIfExpressions=u1>=t1 & u1<t2
  If Action Subsystem1 : Subsystem  TreatAsAtomicUnit=on
  If Action Subsystem2 : Subsystem  TreatAsAtomicUnit=on
  If Action Subsystem3 : Subsystem  TreatAsAtomicUnit=on
  Merge : Merge  Inputs=3
  omega_peak : Outport
  wires:
  Merge/1 -> omega_peak/1
  If Action Subsystem1/1(Out1) -> Merge/1
  If/2 -> If Action Subsystem2/Action
  If Action Subsystem2/1(Out1) -> Merge/2
  If Action Subsystem3/1(Out1) -> Merge/3
  Constant2/1 -> If Action Subsystem3/1(In1)
  Constant/1 -> If Action Subsystem1/1(In1)
  If/1 -> If Action Subsystem1/Action
  If/3 -> If Action Subsystem3/Action
  time/1 -> If/1, If Action Subsystem2/1(In1)

== system GunnerusDP_v1/Environment and Vessel Dynamics/Wave definiton (from MCSim)/wave height and wave frequency/Hs and omega14/hs ==
  time : Inport
  Constant : Constant  Value=v1
  Constant2 : Constant  Value=v2
  If : If  IfExpression=u1 < t1  ElseIfExpressions=u1>=t1 & u1<t2
  If Action Subsystem1 : Subsystem  TreatAsAtomicUnit=on
  If Action Subsystem2 : Subsystem  TreatAsAtomicUnit=on
  If Action Subsystem3 : Subsystem  TreatAsAtomicUnit=on
  Merge : Merge  Inputs=3
  omega_peak : Outport
  wires:
  Merge/1 -> omega_peak/1
  If Action Subsystem1/1(Out1) -> Merge/1
  If/2 -> If Action Subsystem2/Action
  If Action Subsystem2/1(Out1) -> Merge/2
  If Action Subsystem3/1(Out1) -> Merge/3
  Constant2/1 -> If Action Subsystem3/1(In1)
  Constant/1 -> If Action Subsystem1/1(In1)
  If/1 -> If Action Subsystem1/Action
  If/3 -> If Action Subsystem3/Action
  time/1 -> If/1, If Action Subsystem2/1(In1)

== system GunnerusDP_v1/Environment and Vessel Dynamics/Wave definiton (from MCSim)/wave height and wave frequency/Hs and omega14/omega_p ==
  time : Inport
  Constant : Constant  Value=v1
  Constant2 : Constant  Value=v2
  If : If  IfExpression=u1 < t1  ElseIfExpressions=u1>=t1 & u1<t2
  If Action Subsystem1 : Subsystem  TreatAsAtomicUnit=on
  If Action Subsystem2 : Subsystem  TreatAsAtomicUnit=on
  If Action Subsystem3 : Subsystem  TreatAsAtomicUnit=on
  Merge : Merge  Inputs=3
  omega_peak : Outport
  wires:
  time/1 -> If Action Subsystem2/1(In1), If/1
  If/3 -> If Action Subsystem3/Action
  If/1 -> If Action Subsystem1/Action
  Constant/1 -> If Action Subsystem1/1(In1)
  Constant2/1 -> If Action Subsystem3/1(In1)
  If Action Subsystem3/1(Out1) -> Merge/3
  If Action Subsystem2/1(Out1) -> Merge/2
  If/2 -> If Action Subsystem2/Action
  If Action Subsystem1/1(Out1) -> Merge/1
  Merge/1 -> omega_peak/1

== system GunnerusDP_v1/Environment and Vessel Dynamics/Wave definiton (from MCSim)/wave height and wave frequency/Hs and omega15/hs ==
  time : Inport
  Constant : Constant  Value=v1
  Constant2 : Constant  Value=v2
  If : If  IfExpression=u1 < t1  ElseIfExpressions=u1>=t1 & u1<t2
  If Action Subsystem1 : Subsystem  TreatAsAtomicUnit=on
  If Action Subsystem2 : Subsystem  TreatAsAtomicUnit=on
  If Action Subsystem3 : Subsystem  TreatAsAtomicUnit=on
  Merge : Merge  Inputs=3
  omega_peak : Outport
  wires:
  time/1 -> If Action Subsystem2/1(In1), If/1
  If/3 -> If Action Subsystem3/Action
  If/1 -> If Action Subsystem1/Action
  Constant/1 -> If Action Subsystem1/1(In1)
  Constant2/1 -> If Action Subsystem3/1(In1)
  If Action Subsystem3/1(Out1) -> Merge/3
  If Action Subsystem2/1(Out1) -> Merge/2
  If/2 -> If Action Subsystem2/Action
  If Action Subsystem1/1(Out1) -> Merge/1
  Merge/1 -> omega_peak/1

== system GunnerusDP_v1/Environment and Vessel Dynamics/Wave definiton (from MCSim)/wave height and wave frequency/Hs and omega15/omega_p ==
  time : Inport
  Constant : Constant  Value=v1
  Constant2 : Constant  Value=v2
  If : If  IfExpression=u1 < t1  ElseIfExpressions=u1>=t1 & u1<t2
  If Action Subsystem1 : Subsystem  TreatAsAtomicUnit=on
  If Action Subsystem2 : Subsystem  TreatAsAtomicUnit=on
  If Action Subsystem3 : Subsystem  TreatAsAtomicUnit=on
  Merge : Merge  Inputs=3
  omega_peak : Outport
  wires:
  Merge/1 -> omega_peak/1
  If Action Subsystem1/1(Out1) -> Merge/1
  If/2 -> If Action Subsystem2/Action
  If Action Subsystem2/1(Out1) -> Merge/2
  If Action Subsystem3/1(Out1) -> Merge/3
  Constant2/1 -> If Action Subsystem3/1(In1)
  Constant/1 -> If Action Subsystem1/1(In1)
  If/1 -> If Action Subsystem1/Action
  If/3 -> If Action Subsystem3/Action
  time/1 -> If/1, If Action Subsystem2/1(In1)

== system GunnerusDP_v1/Environment and Vessel Dynamics/Wave definiton (from MCSim)/wave height and wave frequency/Hs and omega16/hs ==
  time : Inport
  Constant : Constant  Value=v1
  Constant2 : Constant  Value=v2
  If : If  IfExpression=u1 < t1  ElseIfExpressions=u1>=t1 & u1<t2
  If Action Subsystem1 : Subsystem  TreatAsAtomicUnit=on
  If Action Subsystem2 : Subsystem  TreatAsAtomicUnit=on
  If Action Subsystem3 : Subsystem  TreatAsAtomicUnit=on
  Merge : Merge  Inputs=3
  omega_peak : Outport
  wires:
  time/1 -> If Action Subsystem2/1(In1), If/1
  If/3 -> If Action Subsystem3/Action
  If/1 -> If Action Subsystem1/Action
  Constant/1 -> If Action Subsystem1/1(In1)
  Constant2/1 -> If Action Subsystem3/1(In1)
  If Action Subsystem3/1(Out1) -> Merge/3
  If Action Subsystem2/1(Out1) -> Merge/2
  If/2 -> If Action Subsystem2/Action
  If Action Subsystem1/1(Out1) -> Merge/1
  Merge/1 -> omega_peak/1

== system GunnerusDP_v1/Environment and Vessel Dynamics/Wave definiton (from MCSim)/wave height and wave frequency/Hs and omega16/omega_p ==
  time : Inport
  Constant : Constant  Value=v1
  Constant2 : Constant  Value=v2
  If : If  IfExpression=u1 < t1  ElseIfExpressions=u1>=t1 & u1<t2
  If Action Subsystem1 : Subsystem  TreatAsAtomicUnit=on
  If Action Subsystem2 : Subsystem  TreatAsAtomicUnit=on
  If Action Subsystem3 : Subsystem  TreatAsAtomicUnit=on
  Merge : Merge  Inputs=3
  omega_peak : Outport
  wires:
  Merge/1 -> omega_peak/1
  If Action Subsystem1/1(Out1) -> Merge/1
  If/2 -> If Action Subsystem2/Action
  If Action Subsystem2/1(Out1) -> Merge/2
  If Action Subsystem3/1(Out1) -> Merge/3
  Constant2/1 -> If Action Subsystem3/1(In1)
  Constant/1 -> If Action Subsystem1/1(In1)
  If/1 -> If Action Subsystem1/Action
  If/3 -> If Action Subsystem3/Action
  time/1 -> If/1, If Action Subsystem2/1(In1)

== system GunnerusDP_v1/Environment and Vessel Dynamics/Wave definiton (from MCSim)/wave height and wave frequency/Hs and omega17/hs ==
  time : Inport
  Constant : Constant  Value=v1
  Constant2 : Constant  Value=v2
  If : If  IfExpression=u1 < t1  ElseIfExpressions=u1>=t1 & u1<t2
  If Action Subsystem1 : Subsystem  TreatAsAtomicUnit=on
  If Action Subsystem2 : Subsystem  TreatAsAtomicUnit=on
  If Action Subsystem3 : Subsystem  TreatAsAtomicUnit=on
  Merge : Merge  Inputs=3
  omega_peak : Outport
  wires:
  Merge/1 -> omega_peak/1
  If Action Subsystem1/1(Out1) -> Merge/1
  If/2 -> If Action Subsystem2/Action
  If Action Subsystem2/1(Out1) -> Merge/2
  If Action Subsystem3/1(Out1) -> Merge/3
  Constant2/1 -> If Action Subsystem3/1(In1)
  Constant/1 -> If Action Subsystem1/1(In1)
  If/1 -> If Action Subsystem1/Action
  If/3 -> If Action Subsystem3/Action
  time/1 -> If/1, If Action Subsystem2/1(In1)

== system GunnerusDP_v1/Environment and Vessel Dynamics/Wave definiton (from MCSim)/wave height and wave frequency/Hs and omega17/omega_p ==
  time : Inport
  Constant : Constant  Value=v1
  Constant2 : Constant  Value=v2
  If : If  IfExpression=u1 < t1  ElseIfExpressions=u1>=t1 & u1<t2
  If Action Subsystem1 : Subsystem  TreatAsAtomicUnit=on
  If Action Subsystem2 : Subsystem  TreatAsAtomicUnit=on
  If Action Subsystem3 : Subsystem  TreatAsAtomicUnit=on
  Merge : Merge  Inputs=3
  omega_peak : Outport
  wires:
  time/1 -> If Action Subsystem2/1(In1), If/1
  If/3 -> If Action Subsystem3/Action
  If/1 -> If Action Subsystem1/Action
  Constant/1 -> If Action Subsystem1/1(In1)
  Constant2/1 -> If Action Subsystem3/1(In1)
  If Action Subsystem3/1(Out1) -> Merge/3
  If Action Subsystem2/1(Out1) -> Merge/2
  If/2 -> If Action Subsystem2/Action
  If Action Subsystem1/1(Out1) -> Merge/1
  Merge/1 -> omega_peak/1

== system GunnerusDP_v1/Environment and Vessel Dynamics/Wave definiton (from MCSim)/wave height and wave frequency/Hs and omega18/hs ==
  time : Inport
  Constant : Constant  Value=v1
  Constant2 : Constant  Value=v2
  If : If  IfExpression=u1 < t1  ElseIfExpressions=u1>=t1 & u1<t2
  If Action Subsystem1 : Subsystem  TreatAsAtomicUnit=on
  If Action Subsystem2 : Subsystem  TreatAsAtomicUnit=on
  If Action Subsystem3 : Subsystem  TreatAsAtomicUnit=on
  Merge : Merge  Inputs=3
  omega_peak : Outport
  wires:
  time/1 -> If Action Subsystem2/1(In1), If/1
  If/3 -> If Action Subsystem3/Action
  If/1 -> If Action Subsystem1/Action
  Constant/1 -> If Action Subsystem1/1(In1)
  Constant2/1 -> If Action Subsystem3/1(In1)
  If Action Subsystem3/1(Out1) -> Merge/3
  If Action Subsystem2/1(Out1) -> Merge/2
  If/2 -> If Action Subsystem2/Action
  If Action Subsystem1/1(Out1) -> Merge/1
  Merge/1 -> omega_peak/1

== system GunnerusDP_v1/Environment and Vessel Dynamics/Wave definiton (from MCSim)/wave height and wave frequency/Hs and omega18/omega_p ==
  time : Inport
  Constant : Constant  Value=v1
  Constant2 : Constant  Value=v2
  If : If  IfExpression=u1 < t1  ElseIfExpressions=u1>=t1 & u1<t2
  If Action Subsystem1 : Subsystem  TreatAsAtomicUnit=on
  If Action Subsystem2 : Subsystem  TreatAsAtomicUnit=on
  If Action Subsystem3 : Subsystem  TreatAsAtomicUnit=on
  Merge : Merge  Inputs=3
  omega_peak : Outport
  wires:
  Merge/1 -> omega_peak/1
  If Action Subsystem1/1(Out1) -> Merge/1
  If/2 -> If Action Subsystem2/Action
  If Action Subsystem2/1(Out1) -> Merge/2
  If Action Subsystem3/1(Out1) -> Merge/3
  Constant2/1 -> If Action Subsystem3/1(In1)
  Constant/1 -> If Action Subsystem1/1(In1)
  If/1 -> If Action Subsystem1/Action
  If/3 -> If Action Subsystem3/Action
  time/1 -> If/1, If Action Subsystem2/1(In1)

== system GunnerusDP_v1/Environment and Vessel Dynamics/Wave definiton (from MCSim)/wave height and wave frequency/Hs and omega19/hs ==
  time : Inport
  Constant : Constant  Value=v1
  Constant2 : Constant  Value=v2
  If : If  IfExpression=u1 < t1  ElseIfExpressions=u1>=t1 & u1<t2
  If Action Subsystem1 : Subsystem  TreatAsAtomicUnit=on
  If Action Subsystem2 : Subsystem  TreatAsAtomicUnit=on
  If Action Subsystem3 : Subsystem  TreatAsAtomicUnit=on
  Merge : Merge  Inputs=3
  omega_peak : Outport
  wires:
  Merge/1 -> omega_peak/1
  If Action Subsystem1/1(Out1) -> Merge/1
  If/2 -> If Action Subsystem2/Action
  If Action Subsystem2/1(Out1) -> Merge/2
  If Action Subsystem3/1(Out1) -> Merge/3
  Constant2/1 -> If Action Subsystem3/1(In1)
  Constant/1 -> If Action Subsystem1/1(In1)
  If/1 -> If Action Subsystem1/Action
  If/3 -> If Action Subsystem3/Action
  time/1 -> If/1, If Action Subsystem2/1(In1)

== system GunnerusDP_v1/Environment and Vessel Dynamics/Wave definiton (from MCSim)/wave height and wave frequency/Hs and omega19/omega_p ==
  time : Inport
  Constant : Constant  Value=v1
  Constant2 : Constant  Value=v2
  If : If  IfExpression=u1 < t1  ElseIfExpressions=u1>=t1 & u1<t2
  If Action Subsystem1 : Subsystem  TreatAsAtomicUnit=on
  If Action Subsystem2 : Subsystem  TreatAsAtomicUnit=on
  If Action Subsystem3 : Subsystem  TreatAsAtomicUnit=on
  Merge : Merge  Inputs=3
  omega_peak : Outport
  wires:
  time/1 -> If Action Subsystem2/1(In1), If/1
  If/3 -> If Action Subsystem3/Action
  If/1 -> If Action Subsystem1/Action
  Constant/1 -> If Action Subsystem1/1(In1)
  Constant2/1 -> If Action Subsystem3/1(In1)
  If Action Subsystem3/1(Out1) -> Merge/3
  If Action Subsystem2/1(Out1) -> Merge/2
  If/2 -> If Action Subsystem2/Action
  If Action Subsystem1/1(Out1) -> Merge/1
  Merge/1 -> omega_peak/1

== system GunnerusDP_v1/Environment and Vessel Dynamics/Wave definiton (from MCSim)/wave height and wave frequency/Hs and omega2/hs ==
  time : Inport
  Constant : Constant  Value=v1
  Constant2 : Constant  Value=v2
  If : If  IfExpression=u1 < t1  ElseIfExpressions=u1>=t1 & u1<t2
  If Action Subsystem1 : Subsystem  TreatAsAtomicUnit=on
  If Action Subsystem2 : Subsystem  TreatAsAtomicUnit=on
  If Action Subsystem3 : Subsystem  TreatAsAtomicUnit=on
  Merge : Merge  Inputs=3
  omega_peak : Outport
  wires:
  Merge/1 -> omega_peak/1
  If Action Subsystem1/1(Out1) -> Merge/1
  If/2 -> If Action Subsystem2/Action
  If Action Subsystem2/1(Out1) -> Merge/2
  If Action Subsystem3/1(Out1) -> Merge/3
  Constant2/1 -> If Action Subsystem3/1(In1)
  Constant/1 -> If Action Subsystem1/1(In1)
  If/1 -> If Action Subsystem1/Action
  If/3 -> If Action Subsystem3/Action
  time/1 -> If/1, If Action Subsystem2/1(In1)

== system GunnerusDP_v1/Environment and Vessel Dynamics/Wave definiton (from MCSim)/wave height and wave frequency/Hs and omega2/omega_p ==
  time : Inport
  Constant : Constant  Value=v1
  Constant2 : Constant  Value=v2
  If : If  IfExpression=u1 < t1  ElseIfExpressions=u1>=t1 & u1<t2
  If Action Subsystem1 : Subsystem  TreatAsAtomicUnit=on
  If Action Subsystem2 : Subsystem  TreatAsAtomicUnit=on
  If Action Subsystem3 : Subsystem  TreatAsAtomicUnit=on
  Merge : Merge  Inputs=3
  omega_peak : Outport
  wires:
  time/1 -> If Action Subsystem2/1(In1), If/1
  If/3 -> If Action Subsystem3/Action
  If/1 -> If Action Subsystem1/Action
  Constant/1 -> If Action Subsystem1/1(In1)
  Constant2/1 -> If Action Subsystem3/1(In1)
  If Action Subsystem3/1(Out1) -> Merge/3
  If Action Subsystem2/1(Out1) -> Merge/2
  If/2 -> If Action Subsystem2/Action
  If Action Subsystem1/1(Out1) -> Merge/1
  Merge/1 -> omega_peak/1
